simulink model "lvtest3"  (Simulink 7.1)
settings: Solver=ode4  StartTime=0.0  StopTime=90  FixedStep=0.01  RelTol=1e-3
values from neighbouring files (symbols this model uses):
  Ctorque = cq(2:5:102,2:5:182)    [lv_cankaofile.m]    (also in lv_demofile3.m)
  cut_in = 3    [lv_cankaofile.m]    (also in lv_demofile.m; lv_demofile1.m; lv_demofile2.m; lv_demofile3.m)
  cut_out = 25    [lv_cankaofile.m]    (also in lv_demofile.m; lv_demofile1.m; lv_demofile2.m; lv_demofile3.m)
  fs = 50    [lv_cankaofile.m]
  Jem = 90    [lv_cankaofile.m]    (also in lv_demofile.m = 97.5; lv_demofile1.m = 97.5; lv_demofile2.m = 97.5; lv_demofile3.m = 97.5)
  Jwt = 9e7    (= 90000000)    [lv_cankaofile.m]    (also in lv_demofile.m = 3275300; lv_demofile1.m = 3275300; lv_demofile2.m = 3275300; lv_demofile3.m = 3275300)
  K = 83    [lv_cankaofile.m]    (also in lv_demofile.m; lv_demofile1.m = 75.76; lv_demofile2.m; lv_demofile3.m = 75.76)
  Lm = 0.0123    [lv_cankaofile.m]
  Lsgm_r = 0.0126    [lv_cankaofile.m]
  Lsgm_s = 0.0125    [lv_cankaofile.m]
  p = 2    [lv_cankaofile.m]
  R = 40    [lv_cankaofile.m]    (also in lv_demofile.m = 38.5; lv_demofile1.m = 38.75; lv_demofile2.m = 38.5; lv_demofile3.m = 38.5)
  ro_air = 1.225    [lv_cankaofile.m]    (also in lv_demofile.m = 1.2236; lv_demofile1.m; lv_demofile2.m = 1.2236; lv_demofile3.m)
  roughness = 600    [lv_cankaofile.m]    (also in lv_demofile1.m; lv_demofile3.m; lv_demofile4.m; lv_demofile5.m)
  Rr = 0.0041    [lv_cankaofile.m]
  Rs = 0.0043    [lv_cankaofile.m]
  steptime = 0.01    [lv_cankaofile.m]    (also in lv_demofile1.m; lv_demofile3.m; lv_demofile4.m; lv_demofile5.m)
  Tact = 0    [lv_cankaofile.m]    (also in lv_demofile.m; lv_demofile1.m; lv_demofile2.m; lv_demofile3.m)
  turb_int = 12    [lv_cankaofile.m]    (also in lv_demofile1.m; lv_demofile3.m; lv_demofile4.m; lv_demofile5.m)
undefined symbols (not defined in the file or in its folder): PP, u0
libraries: wt_blockset_v3 x2
settings Model: Creator=xc  LastModifiedBy=lv

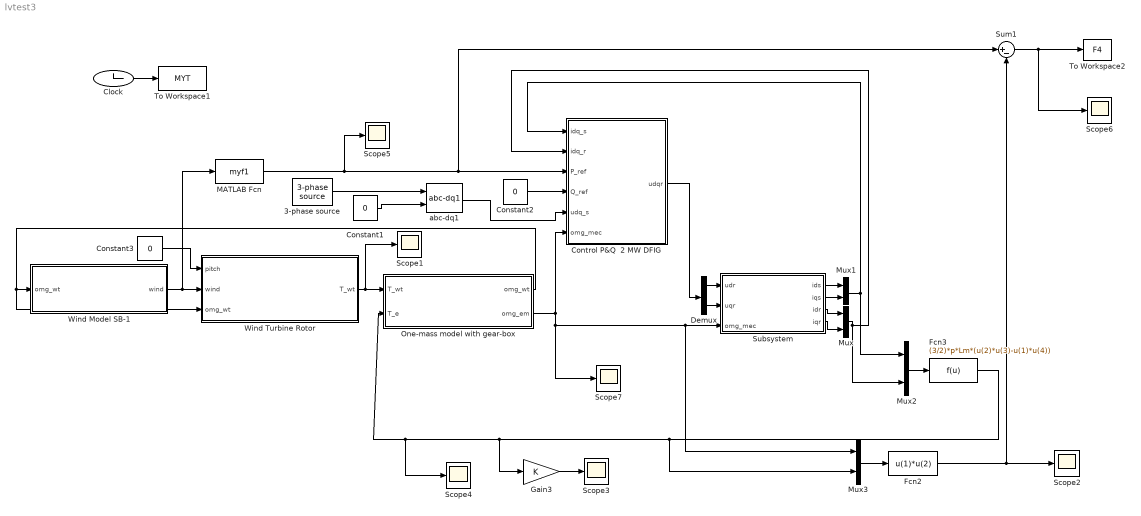
== system lvtest3 ==
  3-phase source : wt_blockset_v3/Grid Models/3-phase source  SystemSampleTime=-1  Uf=220  fs=50
  Clock : Clock
      settings: Decimation=10
  Constant1 : Constant  Value=0  OutDataType=sfix(16)  OutScaling=2^0
  Constant2 : Constant  Value=0  OutDataType=sfix(16)  OutScaling=2^0
  Constant3 : Constant  Value=0  OutDataType=sfix(16)  OutScaling=2^0
  Control P&Q  2 MW DFIG : Subsystem  AncestorBlock="wt_blockset_v3/Control/Control P&Q  2 MW DFIG"  mask(Control P & Q for double feed induction generator){param=[Rs Lsgm_s Rr Lsgm_r Lm], p=p, fs=fs}
      mask prompts: param "Electrical parameters [Rs Lsgm_s Rr Lsgm_r Lm]"; p "Number of pole pais"; fs "Base frequency [Hz]"
      mask help: Control of active and reactive power in synchronous reference frame for DFIG.
      mask init:
      | Rs=param(1); Lsgm_s=param(2); Rr=param(3); Lsgm_r=param(4);
      | Lm=param(5); Lss=Lsgm_s+Lm; Lrr=Lsgm_r+Lm; D=Lss*Lrr-Lm^2;
      | T=D/Lss; Tpr=(Lm^2)/Lss;
      | tau_1=T/Rr;  tau_2=Rr;
      mask Display: disp('Control\nP&Q')
  Demux : Demux  Outputs=2
  Fcn2 : Fcn  Expr=u(1)*u(2)
  Fcn3 : Fcn  Expr=(3/2)*p*Lm*(u(2)*u(3)-u(1)*u(4))
  Gain3 : Gain  Gain=K  ParameterDataType=sfix(16)  ParameterScaling=2^0  OutDataType=sfix(16)  OutScaling=2^0  SaturateOnIntegerOverflow=on  OutDataTypeStr=Inherit: Same as input  ParamDataTypeStr=Inherit: Same as input
  MATLAB Fcn : MATLABFcn  MATLABFcn=myf1
  Mux{,1..3} (4 alike) : Mux  Inputs=2
  One-mass model with gear-box : Subsystem  AncestorBlock=wt_blockset_v3/Mechanical Components/One-mass model with gear-box  mask(Simple Gearbox){Jem=Jem, Jwt=Jwt, K=K, init_speed=1.514}
      mask prompts: Jem "Electric machinery - Moment of inertia [kg m2]"; Jwt "Wind turbine rotor - Moment of inertia [kg*m2]"; K "Gearbox ratio"; init_speed "Initial condition [omg_wt (rad/sec)]"
      mask init:
      | J=Jem*K^2+Jwt;
      mask Display: disp('E M\nGear box')
  Scope{1..7} (7 alike) : Scope
      Scope1 settings: YMin=-2.25e+010  YMax=1.5e+010
      Scope2 settings: TimeRange=90  YMin=-8e+006  YMax=8e+006
      Scope3 settings: YMin=200000  YMax=2.4e+006  SaveName=ScopeData12
      Scope4 settings: YMin=-2.25e+010  YMax=1.5e+010  SaveName=ScopeData6
      Scope5 settings: YMin=-2.25e+010  YMax=1.5e+010  SaveName=ScopeData4
      Scope6 settings: TimeRange=100  YMin=-9e+006  YMax=9e+006  SaveName=ScopeData27
      Scope7 settings: TimeRange=100  YMin=120  YMax=190  SaveName=ScopeData13
  Subsystem : Subsystem
  Sum1 : Sum  Inputs=|+-  OutDataType=sfix(16)  OutScaling=2^0  SaturateOnIntegerOverflow=on  InputSameDT=on  OutDataTypeStr=Inherit: Same as first input
  To Workspace1 : ToWorkspace  VariableName=MYT  SampleTime=-1  SaveFormat=Array
  To Workspace2 : ToWorkspace  VariableName=F4  SampleTime=-1  SaveFormat=Array
  Wind Model SB-1 : Subsystem  AncestorBlock=wt_blockset_v3/Mechanical Components/Wind Model SB-1  TreatAsAtomicUnit=on  mask(Wind Model using Simulink Band-limited white noise generator){D_rotor=2*R, v_mean=10, roughness=roughness, turb_int=turb_int, T_sample=steptime}
      mask prompts: D_rotor "Rotor diameter [m]"; v_mean "Average wind speed [m/sec]"; roughness "Length scale [m]"; turb_int "Turbulence intensity [%]"; T_sample "Sample time [sec]"
      mask help:
      | Implements a rotor wind model developped by RISOE National Laboratory based on Kaimal spectra. The model takes into account the rotational turbulences and the tower shadow.
      | This model uses the built-in band-limited white noise generator from Simulink with different seeds.
      mask init:
      | r = D_rotor/2;
      | sigma = v_mean*turb_int/100;
      | var = sigma^2;
      | c = roughness/(2*pi*v_mean);
      | d = r/v_mean;
      | trans=sigma*sqrt(roughness/v_mean);
      | random=[256, 894, 31];
      mask Display: disp('Wind\nModel\n(SB-1)')
  Wind Turbine Rotor : Subsystem  AncestorBlock=wt_blockset_beta/Mechanical Components/Wind Turbine Rotor  mask(Aerodynamic model for wind turbine){R=R, ro_air=ro_air, cut_in=cut_in, cut_out=cut_out, Tact=Tact}
      mask prompts: R "Blade radius [m]"; ro_air "Air density [kg m3]"; cut_in "Cut in speed [m/sec]"; cut_out "Cut out speed [m/sec]"; Tact "Time constant for pitch actuator [sec]"
      mask init:
      | %cq_table
      mask Display: plot(20,0,120,200,[45,35,35,45,75,75,45],[85,92,108,115,115,85,85],[55,50,70,65],[115,180,190,115],[55,50,70,65],[85,10,20,85],[75,85],[102,102],[75,85],[98,98],[105,85,85,105],[80,85,115,120])
  abc-dq1 : wt_blockset_v3/Electrical Machinery/Simulink Blocks  based Models/Wound Rotor Induction Machine constant parameters/abc-dq1  SystemSampleTime=-1
  wires:
  MATLAB Fcn/1 -> Scope5/1, Sum1/1, Control P&Q  2 MW DFIG/3(P_ref)
  Constant2/1 -> Control P&Q  2 MW DFIG/4(Q_ref)
  Subsystem/1(ids) -> Mux1/1
  Subsystem/2(iqs) -> Mux1/2
  Mux1/1 -> Mux2/1, Control P&Q  2 MW DFIG/1(idq_s)
  Subsystem/3(idr) -> Mux/1
  Subsystem/4(iqr) -> Mux/2
  Mux/1 -> Mux2/2, Control P&Q  2 MW DFIG/2(idq_r)
  Control P&Q  2 MW DFIG/1(udqr) -> Demux/1
  Demux/1 -> Subsystem/1(udr)
  Demux/2 -> Subsystem/2(uqr)
  Wind Turbine Rotor/1(T_wt) -> One-mass model with gear-box/1(T_wt), Scope1/1
  Constant3/1 -> Wind Turbine Rotor/1(pitch)
  Wind Model SB-1/1(wind) -> Wind Turbine Rotor/2(wind), MATLAB Fcn/1
  One-mass model with gear-box/1(omg_wt) -> Wind Model SB-1/1(omg_wt), Wind Turbine Rotor/3(omg_wt)
  Mux2/1 -> Fcn3/1
  Fcn3/1 -> Gain3/1, One-mass model with gear-box/2(T_e), Scope4/1, Mux3/2
  Gain3/1 -> Scope3/1
  Mux3/1 -> Fcn2/1
  Fcn2/1 -> Scope2/1, Sum1/2
  One-mass model with gear-box/2(omg_em) -> Control P&Q  2 MW DFIG/6(omg_mec), Subsystem/3(omg_mec), Mux3/1, Scope7/1
  Clock/1 -> To Workspace1/1
  Sum1/1 -> To Workspace2/1, Scope6/1
  3-phase source/1 -> abc-dq1/1
  Constant1/1 -> abc-dq1/2
  abc-dq1/1 -> Control P&Q  2 MW DFIG/5(udq_s)

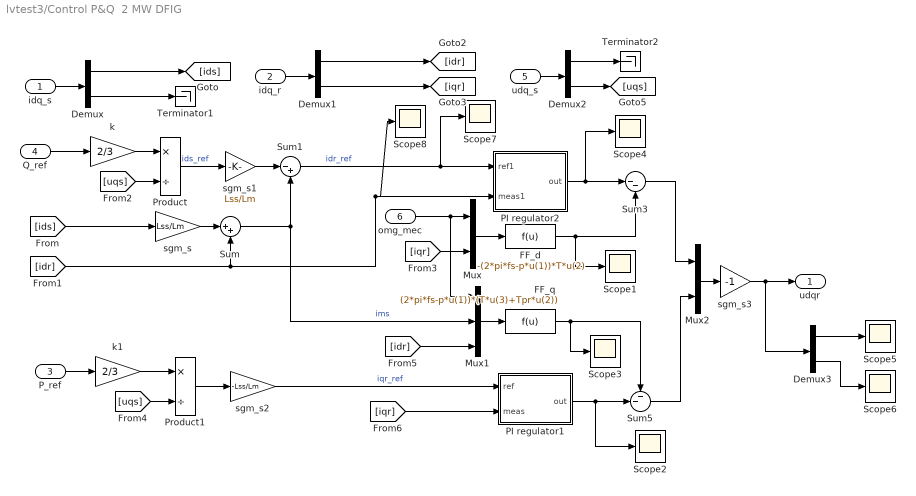
== system lvtest3/Control P&Q  2 MW DFIG ==
  idq_s : Inport  OutDataType=sfix(16)  OutScaling=2^0
  idq_r : Inport  Port=2  OutDataType=sfix(16)  OutScaling=2^0
  P_ref : Inport  Port=3  OutDataType=sfix(16)  OutScaling=2^0
  Q_ref : Inport  Port=4  OutDataType=sfix(16)  OutScaling=2^0
  udq_s : Inport  Port=5  OutDataType=sfix(16)  OutScaling=2^0
  omg_mec : Inport  Port=6  OutDataType=sfix(16)  OutScaling=2^0
  Demux{,1..3} (4 alike) : Demux  Outputs=2
  FF_d : Fcn  Expr=-(2*pi*fs-p*u(1))*T*u(2)
  FF_q : Fcn  Expr=(2*pi*fs-p*u(1))*(T*u(3)+Tpr*u(2))
  Mux : Mux  Inputs=2
  Mux1 : Mux  Inputs=3
  Mux2 : Mux  Inputs=2
  PI regulator1 : Subsystem  mask{K=PP(3), Ti=PP(4), ka=10, maxim=100, init_cond=0}
      mask prompts: K "Proportional Constant"; Ti "Integrate constant"; maxim "Limits"; init_cond "initial"
  PI regulator2 : Subsystem  mask{K=PP(1), Ti=PP(2), init_cond=0}
      mask prompts: K "Proportional Constant"; Ti "Integrate constant"; init_cond "initial"
  Product : Product  Inputs=*/  OutDataType=sfix(16)  OutScaling=2^0  SaturateOnIntegerOverflow=on  InputSameDT=on  OutDataTypeStr=Inherit: Same as first input
  Product1 : Product  Inputs=*/  OutDataType=sfix(16)  OutScaling=2^0  SaturateOnIntegerOverflow=on  InputSameDT=on  OutDataTypeStr=Inherit: Same as first input
  Scope{1..8} (8 alike) : Scope
      Scope1 settings: YMin=-2.25e+010  YMax=1.5e+010  SaveName=ScopeData5
      Scope2 settings: YMin=-2.25e+010  YMax=1.5e+010  SaveName=ScopeData7
      Scope3 settings: YMin=-2.25e+010  YMax=1.5e+010  SaveName=ScopeData3
      Scope4 settings: YMin=-125  YMax=150  SaveName=ScopeData8
      Scope5 settings: YMin=-2.25e+010  YMax=1.5e+010  SaveName=ScopeData9
      Scope6 settings: YMin=-2.25e+010  YMax=1.5e+010  SaveName=ScopeData10
      Scope7 settings: YMin=-2.25e+010  YMax=1.5e+010  SaveName=ScopeData28
      Scope8 settings: YMin=-2.25e+010  YMax=1.5e+010  SaveName=ScopeData29
  Sum : Sum  Inputs=|++  OutDataType=sfix(16)  OutScaling=2^0  SaturateOnIntegerOverflow=on  InputSameDT=on  OutDataTypeStr=Inherit: Same as first input
  Sum1 : Sum  Inputs=|-+  OutDataType=sfix(16)  OutScaling=2^0  SaturateOnIntegerOverflow=on  InputSameDT=on  OutDataTypeStr=Inherit: Same as first input
  Sum3 : Sum  Inputs=|--  OutDataType=sfix(16)  OutScaling=2^0  SaturateOnIntegerOverflow=on  InputSameDT=on  OutDataTypeStr=Inherit: Same as first input
  Sum5 : Sum  Inputs=--|  OutDataType=sfix(16)  OutScaling=2^0  SaturateOnIntegerOverflow=on  InputSameDT=on  OutDataTypeStr=Inherit: Same as first input
  Terminator1 : Terminator
  Terminator2 : Terminator
  k : Gain  Gain=2/3  ParameterDataType=sfix(16)  ParameterScaling=2^0  OutDataType=sfix(16)  OutScaling=2^0  SaturateOnIntegerOverflow=on  OutDataTypeStr=Inherit: Same as input  ParamDataTypeStr=Inherit: Same as input
  k1 : Gain  Gain=2/3  ParameterDataType=sfix(16)  ParameterScaling=2^0  OutDataType=sfix(16)  OutScaling=2^0  SaturateOnIntegerOverflow=on  OutDataTypeStr=Inherit: Same as input  ParamDataTypeStr=Inherit: Same as input
  sgm_s : Gain  Gain=Lss/Lm  ParameterDataType=sfix(16)  ParameterScaling=2^0  OutDataType=sfix(16)  OutScaling=2^0  SaturateOnIntegerOverflow=on  OutDataTypeStr=Inherit: Same as input  ParamDataTypeStr=Inherit: Same as input
  sgm_s1 : Gain  Gain=Lss/Lm  ParameterDataType=sfix(16)  ParameterScaling=2^0  OutDataType=sfix(16)  OutScaling=2^0  SaturateOnIntegerOverflow=on  OutDataTypeStr=Inherit: Same as input  ParamDataTypeStr=Inherit: Same as input
  sgm_s2 : Gain  Gain=-Lss/Lm  ParameterDataType=sfix(16)  ParameterScaling=2^0  OutDataType=sfix(16)  OutScaling=2^0  SaturateOnIntegerOverflow=on  OutDataTypeStr=Inherit: Same as input  ParamDataTypeStr=Inherit: Same as input
  sgm_s3 : Gain  Gain=-1  ParameterDataType=sfix(16)  ParameterScaling=2^0  OutDataType=sfix(16)  OutScaling=2^0  SaturateOnIntegerOverflow=on  OutDataTypeStr=Inherit: Same as input  ParamDataTypeStr=Inherit: Same as input
  udqr : Outport  OutDataType=sfix(16)  OutScaling=2^0
  wires:
  idq_s/1 -> Demux/1
  idq_r/1 -> Demux1/1
  Demux/1 -> [ids]
  Demux/2 -> Terminator1/1
  Demux1/2 -> [iqr]
  [ids] -> sgm_s/1
  sgm_s/1 -> Sum/1
  [idr] -> Sum/2, PI regulator2/2(meas1), Scope8/1
  udq_s/1 -> Demux2/1
  Demux2/1 -> Terminator2/1
  Demux2/2 -> [uqs]
  Q_ref/1 -> k/1
  k/1 -> Product/1
  [uqs] -> Product/2
  Product/1 -> sgm_s1/1  "ids_ref"
  Sum/1 -> Sum1/2, Mux1/2  "ims"
  PI regulator2/1(out) -> Sum3/1, Scope4/1
  omg_mec/1 -> Mux/1, Mux1/1
  Mux/1 -> FF_d/1
  [iqr] -> Mux/2
  Sum3/1 -> Mux2/1
  P_ref/1 -> k1/1
  k1/1 -> Product1/1
  [uqs] -> Product1/2
  Product1/1 -> sgm_s2/1
  sgm_s2/1 -> PI regulator1/1(ref)  "iqr_ref"
  Mux1/1 -> FF_q/1
  PI regulator1/1(out) -> Sum5/2, Scope2/1
  [idr] -> Mux1/3
  Sum5/1 -> Mux2/2
  Mux2/1 -> sgm_s3/1
  sgm_s1/1 -> Sum1/1
  Sum1/1 -> PI regulator2/1(ref1), Scope7/1  "idr_ref"
  FF_d/1 -> Sum3/2, Scope1/1
  [iqr] -> PI regulator1/2(meas)
  FF_q/1 -> Scope3/1, Sum5/1
  Demux1/1 -> [idr]
  Demux3/1 -> Scope5/1
  Demux3/2 -> Scope6/1
  sgm_s3/1 -> udqr/1, Demux3/1

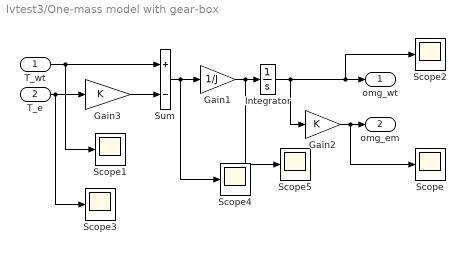
== system lvtest3/One-mass model with gear-box ==
  T_wt : Inport  OutDataType=sfix(16)  OutScaling=2^0
  T_e : Inport  Port=2  OutDataType=sfix(16)  OutScaling=2^0
  Gain1 : Gain  Gain=1/J  ParameterDataType=sfix(16)  ParameterScaling=2^0  OutDataType=sfix(16)  OutScaling=2^0  SaturateOnIntegerOverflow=on  OutDataTypeStr=Inherit: Same as input  ParamDataTypeStr=Inherit: Same as input
  Gain2 : Gain  Gain=K  ParameterDataType=sfix(16)  ParameterScaling=2^0  OutDataType=sfix(16)  OutScaling=2^0  SaturateOnIntegerOverflow=on  OutDataTypeStr=Inherit: Same as input  ParamDataTypeStr=Inherit: Same as input
  Gain3 : Gain  Gain=K  ParameterDataType=sfix(16)  ParameterScaling=2^0  OutDataType=sfix(16)  OutScaling=2^0  SaturateOnIntegerOverflow=on  OutDataTypeStr=Inherit: Same as input  ParamDataTypeStr=Inherit: Same as input
  Integrator : Integrator  InitialCondition=init_speed  UpperSaturationLimit=0.95*2*pi*60  LowerSaturationLimit=0
  Scope{,1..5} (6 alike) : Scope
      Scope settings: TimeRange=10  SaveName=ScopeData20
      Scope1 settings: TimeRange=10  SaveName=ScopeData24
      Scope2 settings: YMin=-2.25e+010  YMax=1.5e+010  SaveName=ScopeData21
      Scope3 settings: TimeRange=10  SaveName=ScopeData25
      Scope4 settings: TimeRange=10  SaveName=ScopeData2
      Scope5 settings: TimeRange=10  SaveName=ScopeData22
  Sum : Sum  Inputs=+-  OutDataType=sfix(16)  OutScaling=2^0  SaturateOnIntegerOverflow=on  InputSameDT=on  OutDataTypeStr=Inherit: Same as first input
  omg_wt : Outport  OutDataType=sfix(16)  OutScaling=2^0  InitialOutput=0
  omg_em : Outport  Port=2  OutDataType=sfix(16)  OutScaling=2^0  InitialOutput=0
  wires:
  Gain3/1 -> Sum/2
  Gain2/1 -> omg_em/1, Scope/1
  Integrator/1 -> Gain2/1, omg_wt/1, Scope2/1
  T_wt/1 -> Sum/1, Scope1/1
  T_e/1 -> Gain3/1, Scope3/1
  Sum/1 -> Gain1/1, Scope4/1
  Gain1/1 -> Integrator/1, Scope5/1

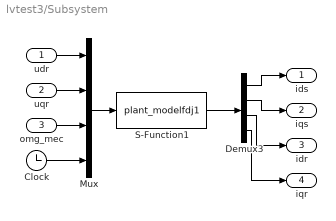
== system lvtest3/Subsystem ==
  udr : Inport
  uqr : Inport  Port=2
  omg_mec : Inport  Port=3
  Clock : Clock
      settings: Decimation=10
  Demux3 : Demux
  Mux : Mux
  S-Function1 : S-Function  FunctionName=plant_modelfdj1  EnableBusSupport=off
  ids : Outport  OutDataType=sfix(16)  OutScaling=2^0  InitialOutput=0
  iqs : Outport  Port=2  OutDataType=sfix(16)  OutScaling=2^0  InitialOutput=0
  idr : Outport  Port=3  OutDataType=sfix(16)  OutScaling=2^0  InitialOutput=0
  iqr : Outport  Port=4  OutDataType=sfix(16)  OutScaling=2^0  InitialOutput=0
  wires:
  Mux/1 -> S-Function1/1
  udr/1 -> Mux/1
  S-Function1/1 -> Demux3/1
  omg_mec/1 -> Mux/3
  uqr/1 -> Mux/2
  Demux3/1 -> ids/1
  Demux3/2 -> iqs/1
  Demux3/3 -> idr/1
  Demux3/4 -> iqr/1
  Clock/1 -> Mux/4

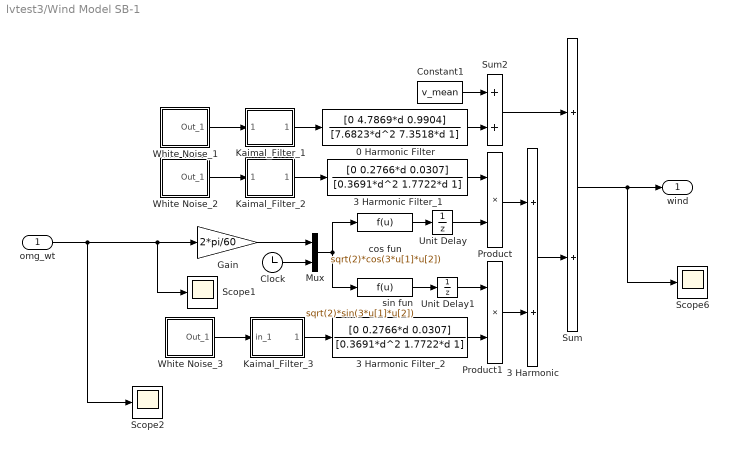
== system lvtest3/Wind Model SB-1 ==
  omg_wt : Inport  OutDataType=sfix(16)  OutScaling=2^0
  0 Harmonic Filter : TransferFcn  Numerator=[0 4.7869*d 0.9904]  Denominator=[7.6823*d^2 7.3518*d 1]
  3 Harmonic : Sum  OutDataType=sfix(16)  OutScaling=2^0  SaturateOnIntegerOverflow=on  InputSameDT=on  OutDataTypeStr=Inherit: Same as first input
  3 Harmonic Filter_1 : TransferFcn  Numerator=[0 0.2766*d 0.0307]  Denominator=[0.3691*d^2 1.7722*d 1]
  3 Harmonic Filter_2 : TransferFcn  Numerator=[0 0.2766*d 0.0307]  Denominator=[0.3691*d^2 1.7722*d 1]
  Clock : Clock
  Constant1 : Constant  Value=v_mean  OutDataType=sfix(16)  OutScaling=2^0
  Gain : Gain  Gain=2*pi/60  ParameterDataType=sfix(16)  ParameterScaling=2^0  OutDataType=sfix(16)  OutScaling=2^0  SaturateOnIntegerOverflow=on  OutDataTypeStr=Inherit: Same as input  ParamDataTypeStr=Inherit: Same as input
  Kaimal_Filter_1 : Subsystem
  Kaimal_Filter_2 : Subsystem
  Kaimal_Filter_3 : Subsystem
  Mux : Mux  Inputs=2
  Product : Product  OutDataType=sfix(16)  OutScaling=2^0  SaturateOnIntegerOverflow=on  InputSameDT=on  OutDataTypeStr=Inherit: Same as first input
  Product1 : Product  OutDataType=sfix(16)  OutScaling=2^0  SaturateOnIntegerOverflow=on  InputSameDT=on  OutDataTypeStr=Inherit: Same as first input
  Scope1 : Scope
      settings: YMin=-2.25e+010  YMax=1.5e+010  SaveName=ScopeData22
  Scope2 : Scope
      settings: YMin=-2.25e+010  YMax=1.5e+010  SaveName=ScopeData20
  Scope6 : Scope
      settings: TimeRange=100  YMin=-9e+006  YMax=9e+006  SaveName=ScopeData39
  Sum : Sum  OutDataType=sfix(16)  OutScaling=2^0  SaturateOnIntegerOverflow=on  InputSameDT=on  OutDataTypeStr=Inherit: Same as first input
  Sum2 : Sum  OutDataType=sfix(16)  OutScaling=2^0  SaturateOnIntegerOverflow=on  InputSameDT=on  OutDataTypeStr=Inherit: Same as first input
  Unit Delay : UnitDelay  SampleTime=T_sample
  Unit Delay1 : UnitDelay  SampleTime=T_sample
  White Noise_1 : Subsystem  mask(Continuous White Noise.){Cov=[1], Ts=T_sample, seed=[random(1)]}
      mask prompts: Cov "Noise Power:"; Ts "Sample Time:"
      mask help:
      | White noise for continuous (s-domain) systems.
      | Band-limited using zero-order-hold.
      mask init:
      | r = rand(1,12); r2 = [r(1),r;r,r(12)]; t =[1:13;1:13];
      mask Help: Implemented using white noise into Zero-Order Hold block. The seed and power can be vectors of the same length to produce a vector of white noise sources. For faster simulation, set sample time to the highest value possible but in accordance with the fastest dynamics of system.
      mask Display: plot(t(:),r2(:))
  White Noise_2 : Subsystem  mask(Continuous White Noise.){@1=[1], @2=T_sample, @3=[random(2)]}
      mask prompts: @1 "Noise Power:"; @2 "Sample Time:"; @3 "Seed"
      mask help:
      | White noise for continuous (s-domain) systems.
      | Band-limited using zero-order-hold.
      mask init:
      | Cov = @1; Ts = @2; seed = @3; r = rand(1,12); r2 = [r(1),r;r,r(12)]; t =[1:13;1:13];
      mask Help: Implemented using white noise into Zero-Order Hold block. The seed and power can be vectors of the same length to produce a vector of white noise sources. For faster simulation, set sample time to the highest value possible but in accordance with the fastest dynamics of system.
      mask Display: plot(t(:),r2(:))
  White Noise_3 : Subsystem  mask(Continuous White Noise.){@1=[1], @2=T_sample, @3=[random(3)]}
      mask prompts: @1 "Noise Power:"; @2 "Sample Time:"; @3 "Seed"
      mask help:
      | White noise for continuous (s-domain) systems.
      | Band-limited using zero-order-hold.
      mask init:
      | Cov = @1; Ts = @2; seed = @3; r = rand(1,12); r2 = [r(1),r;r,r(12)]; t =[1:13;1:13];
      mask Help: Implemented using white noise into Zero-Order Hold block. The seed and power can be vectors of the same length to produce a vector of white noise sources. For faster simulation, set sample time to the highest value possible but in accordance with the fastest dynamics of system.
      mask Display: plot(t(:),r2(:))
  cos fun : Fcn  Expr=sqrt(2)*cos(3*u[1]*u[2])
  sin fun : Fcn  Expr=sqrt(2)*sin(3*u[1]*u[2])
  wind : Outport  OutDataType=sfix(16)  OutScaling=2^0  InitialOutput=[u0]
  wires:
  Clock/1 -> Mux/2
  Unit Delay1/1 -> Product1/1
  Unit Delay/1 -> Product/2
  Gain/1 -> Mux/1
  omg_wt/1 -> Gain/1, Scope1/1, Scope2/1
  Mux/1 -> sin fun/1, cos fun/1
  3 Harmonic Filter_1/1 -> Product/1
  White Noise_3/1(Out_1) -> Kaimal_Filter_3/1(in_1)
  White Noise_2/1(Out_1) -> Kaimal_Filter_2/1(in_1)
  White Noise_1/1(Out_1) -> Kaimal_Filter_1/1(in_1)
  Kaimal_Filter_1/1(out_1) -> 0 Harmonic Filter/1
  Sum/1 -> wind/1, Scope6/1
  Constant1/1 -> Sum2/1
  Sum2/1 -> Sum/1
  0 Harmonic Filter/1 -> Sum2/2
  3 Harmonic/1 -> Sum/2
  3 Harmonic Filter_2/1 -> Product1/2
  Product1/1 -> 3 Harmonic/2
  Product/1 -> 3 Harmonic/1
  sin fun/1 -> Unit Delay1/1
  cos fun/1 -> Unit Delay/1
  Kaimal_Filter_3/1(out_1) -> 3 Harmonic Filter_2/1
  Kaimal_Filter_2/1(out_1) -> 3 Harmonic Filter_1/1

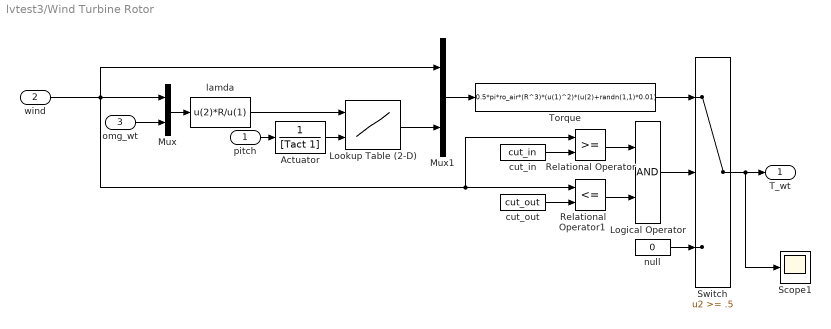
== system lvtest3/Wind Turbine Rotor ==
  pitch : Inport  OutDataType=sfix(16)  OutScaling=2^0
  wind : Inport  Port=2  OutDataType=sfix(16)  OutScaling=2^0
  omg_wt : Inport  Port=3  OutDataType=sfix(16)  OutScaling=2^0
  Actuator : TransferFcn  Denominator=[Tact 1]
  Logical Operator : Logic
  Lookup Table (2-D) : Lookup2D  RowIndex=[0:1:20]  ColumnIndex=[-90:5:90]  Table=Ctorque  OutDataType=sfix(16)  OutScaling=2^0
  Mux : Mux  Inputs=2
  Mux1 : Mux  Inputs=2
  Relational Operator : RelationalOperator  InputSameDT=on
  Relational Operator1 : RelationalOperator  Operator=<=  InputSameDT=on
  Scope1 : Scope
      settings: TimeRange=20  YMin=-1500000  YMax=1500000  SaveName=ScopeData19
  Switch : Switch  Threshold=.5  SaturateOnIntegerOverflow=on  InputSameDT=on
  Torque : Fcn  Expr=0.5*pi*ro_air*(R^3)*(u(1)^2)*(u(2)+randn(1,1)*0.01)
  cut_in : Constant  Value=cut_in  OutDataType=sfix(16)  OutScaling=2^0
  cut_out : Constant  Value=cut_out  OutDataType=sfix(16)  OutScaling=2^0
  lamda : Fcn  Expr=u(2)*R/u(1)
  null : Constant  Value=0  OutDataType=sfix(16)  OutScaling=2^0
  T_wt : Outport
  wires:
  Actuator/1 -> Lookup Table (2-D)/2
  Mux/1 -> lamda/1
  Mux1/1 -> Torque/1
  omg_wt/1 -> Mux/2
  cut_in/1 -> Relational Operator/2
  cut_out/1 -> Relational Operator1/2
  Relational Operator1/1 -> Logical Operator/2
  Relational Operator/1 -> Logical Operator/1
  Switch/1 -> T_wt/1, Scope1/1
  Torque/1 -> Switch/1
  null/1 -> Switch/3
  Logical Operator/1 -> Switch/2
  wind/1 -> Mux/1, Relational Operator/1, Relational Operator1/1, Mux1/1
  Lookup Table (2-D)/1 -> Mux1/2
  lamda/1 -> Lookup Table (2-D)/1
  pitch/1 -> Actuator/1

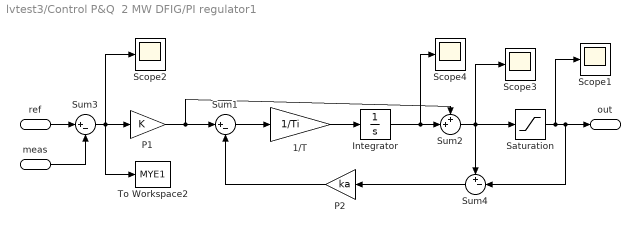
== system lvtest3/Control P&Q  2 MW DFIG/PI regulator1 ==
  ref : Inport  OutDataType=sfix(16)  OutScaling=2^0
  meas : Inport  Port=2  OutDataType=sfix(16)  OutScaling=2^0
  1/T : Gain  Gain=1/Ti  ParameterDataType=sfix(16)  ParameterScaling=2^0  OutDataType=sfix(16)  OutScaling=2^0  SaturateOnIntegerOverflow=on  OutDataTypeStr=Inherit: Same as input  ParamDataTypeStr=Inherit: Same as input
  Integrator : Integrator  InitialCondition=init_cond
  P1 : Gain  Gain=K  ParameterDataType=sfix(16)  ParameterScaling=2^0  OutDataType=sfix(16)  OutScaling=2^0  SaturateOnIntegerOverflow=on  OutDataTypeStr=Inherit: Same as input  ParamDataTypeStr=Inherit: Same as input
  P2 : Gain  Orientation=left  Gain=ka  ParameterDataType=sfix(16)  ParameterScaling=2^0  OutDataType=sfix(16)  OutScaling=2^0  SaturateOnIntegerOverflow=on  OutDataTypeStr=Inherit: Same as input  ParamDataTypeStr=Inherit: Same as input
  Saturation : Saturate  UpperLimit=maxim  LowerLimit=-maxim
  Scope{1..4} (4 alike) : Scope
      Scope1 settings: YMin=-45000  YMax=55000  SaveName=ScopeData30
      Scope2 settings: YMin=-2.25e+010  YMax=1.5e+010  SaveName=ScopeData18
      Scope3 settings: YMin=-2.25e+010  YMax=1.5e+010  SaveName=ScopeData31
      Scope4 settings: YMin=-2.25e+010  YMax=1.5e+010  SaveName=ScopeData34
  Sum1 : Sum  Inputs=|+-  OutDataType=sfix(16)  OutScaling=2^0  SaturateOnIntegerOverflow=on  InputSameDT=on  OutDataTypeStr=Inherit: Same as first input
  Sum2 : Sum  Inputs=++|  OutDataType=sfix(16)  OutScaling=2^0  SaturateOnIntegerOverflow=on  InputSameDT=on  OutDataTypeStr=Inherit: Same as first input
  Sum3 : Sum  Inputs=|+-  OutDataType=sfix(16)  OutScaling=2^0  SaturateOnIntegerOverflow=on  InputSameDT=on  OutDataTypeStr=Inherit: Same as first input
  Sum4 : Sum  Orientation=left  Inputs=+-|  OutDataType=sfix(16)  OutScaling=2^0  SaturateOnIntegerOverflow=on  InputSameDT=on  OutDataTypeStr=Inherit: Same as first input
  To Workspace2 : ToWorkspace  VariableName=MYE1  SampleTime=-1  SaveFormat=Array
  out : Outport  OutDataType=sfix(16)  OutScaling=2^0  InitialOutput=0
  wires:
  Sum2/1 -> Scope3/1, Sum4/1, Saturation/1
  meas/1 -> Sum3/2
  P1/1 -> Sum2/1, Sum1/1
  ref/1 -> Sum3/1
  Sum3/1 -> P1/1, To Workspace2/1, Scope2/1
  1/T/1 -> Integrator/1
  Integrator/1 -> Sum2/2, Scope4/1
  Sum1/1 -> 1/T/1
  P2/1 -> Sum1/2
  Sum4/1 -> P2/1
  Saturation/1 -> Scope1/1, Sum4/2, out/1

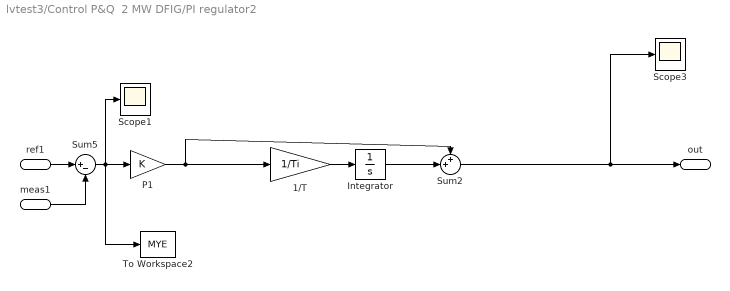
== system lvtest3/Control P&Q  2 MW DFIG/PI regulator2 ==
  ref1 : Inport  OutDataType=sfix(16)  OutScaling=2^0
  meas1 : Inport  Port=2  OutDataType=sfix(16)  OutScaling=2^0
  1/T : Gain  Gain=1/Ti  ParameterDataType=sfix(16)  ParameterScaling=2^0  OutDataType=sfix(16)  OutScaling=2^0  SaturateOnIntegerOverflow=on  OutDataTypeStr=Inherit: Same as input  ParamDataTypeStr=Inherit: Same as input
  Integrator : Integrator  InitialCondition=init_cond
  P1 : Gain  Gain=K  ParameterDataType=sfix(16)  ParameterScaling=2^0  OutDataType=sfix(16)  OutScaling=2^0  SaturateOnIntegerOverflow=on  OutDataTypeStr=Inherit: Same as input  ParamDataTypeStr=Inherit: Same as input
  Scope1 : Scope
      settings: YMin=-4000  YMax=4000  SaveName=ScopeData16
  Scope3 : Scope
      settings: YMin=-7500  YMax=17500  SaveName=ScopeData38
  Sum2 : Sum  Inputs=++|  OutDataType=sfix(16)  OutScaling=2^0  SaturateOnIntegerOverflow=on  InputSameDT=on  OutDataTypeStr=Inherit: Same as first input
  Sum5 : Sum  Inputs=|+-  OutDataType=sfix(16)  OutScaling=2^0  SaturateOnIntegerOverflow=on  InputSameDT=on  OutDataTypeStr=Inherit: Same as first input
  To Workspace2 : ToWorkspace  VariableName=MYE  SampleTime=-1  SaveFormat=Array
  out : Outport  OutDataType=sfix(16)  OutScaling=2^0  InitialOutput=0
  wires:
  Sum2/1 -> out/1, Scope3/1
  P1/1 -> Sum2/1, 1/T/1
  Sum5/1 -> P1/1, To Workspace2/1, Scope1/1
  1/T/1 -> Integrator/1
  Integrator/1 -> Sum2/2
  meas1/1 -> Sum5/2
  ref1/1 -> Sum5/1

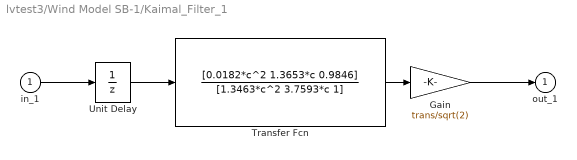
== system lvtest3/Wind Model SB-1/Kaimal_Filter_1 ==
  in_1 : Inport  OutDataType=sfix(16)  OutScaling=2^0
  Gain : Gain  Gain=trans/sqrt(2)  ParameterDataType=sfix(16)  ParameterScaling=2^0  OutDataType=sfix(16)  OutScaling=2^0  SaturateOnIntegerOverflow=on  OutDataTypeStr=Inherit: Same as input  ParamDataTypeStr=Inherit: Same as input
  Transfer Fcn : TransferFcn  Numerator=[0.0182*c^2 1.3653*c 0.9846]  Denominator=[1.3463*c^2 3.7593*c 1]
  Unit Delay : UnitDelay  SampleTime=T_sample
  out_1 : Outport  OutDataType=sfix(16)  OutScaling=2^0
  wires:
  Transfer Fcn/1 -> Gain/1
  in_1/1 -> Unit Delay/1
  Gain/1 -> out_1/1
  Unit Delay/1 -> Transfer Fcn/1

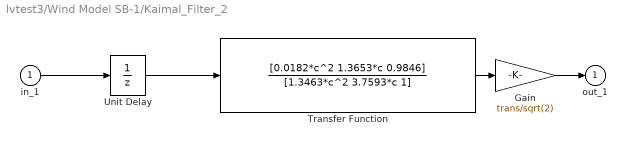
== system lvtest3/Wind Model SB-1/Kaimal_Filter_2 ==
  in_1 : Inport  OutDataType=sfix(16)  OutScaling=2^0
  Gain : Gain  Gain=trans/sqrt(2)  ParameterDataType=sfix(16)  ParameterScaling=2^0  OutDataType=sfix(16)  OutScaling=2^0  SaturateOnIntegerOverflow=on  OutDataTypeStr=Inherit: Same as input  ParamDataTypeStr=Inherit: Same as input
  Transfer Function : TransferFcn  Numerator=[0.0182*c^2 1.3653*c 0.9846]  Denominator=[1.3463*c^2 3.7593*c 1]
  Unit Delay : UnitDelay  SampleTime=T_sample
  out_1 : Outport  OutDataType=sfix(16)  OutScaling=2^0
  wires:
  Transfer Function/1 -> Gain/1
  in_1/1 -> Unit Delay/1
  Gain/1 -> out_1/1
  Unit Delay/1 -> Transfer Function/1

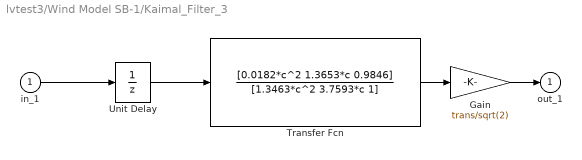
== system lvtest3/Wind Model SB-1/Kaimal_Filter_3 ==
  in_1 : Inport  OutDataType=sfix(16)  OutScaling=2^0
  Gain : Gain  Gain=trans/sqrt(2)  ParameterDataType=sfix(16)  ParameterScaling=2^0  OutDataType=sfix(16)  OutScaling=2^0  SaturateOnIntegerOverflow=on  OutDataTypeStr=Inherit: Same as input  ParamDataTypeStr=Inherit: Same as input
  Transfer Fcn : TransferFcn  Numerator=[0.0182*c^2 1.3653*c 0.9846]  Denominator=[1.3463*c^2 3.7593*c 1]
  Unit Delay : UnitDelay  SampleTime=T_sample
  out_1 : Outport  OutDataType=sfix(16)  OutScaling=2^0
  wires:
  Transfer Fcn/1 -> Gain/1
  in_1/1 -> Unit Delay/1
  Gain/1 -> out_1/1
  Unit Delay/1 -> Transfer Fcn/1

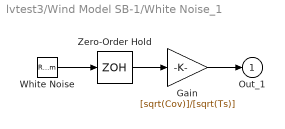
== system lvtest3/Wind Model SB-1/White Noise_1 ==
  Gain : Gain  Gain=[sqrt(Cov)]/[sqrt(Ts)]  ParameterDataType=sfix(16)  ParameterScaling=2^0  OutDataType=sfix(16)  OutScaling=2^0  SaturateOnIntegerOverflow=on  OutDataTypeStr=Inherit: Same as input  ParamDataTypeStr=Inherit: Same as input
  White Noise : RandomNumber  Seed=seed  SampleTime=Ts
  Zero-Order Hold : ZeroOrderHold  SampleTime=Ts
  Out_1 : Outport  OutDataType=sfix(16)  OutScaling=2^0
  wires:
  Zero-Order Hold/1 -> Gain/1
  Gain/1 -> Out_1/1
  White Noise/1 -> Zero-Order Hold/1

== system lvtest3/Wind Model SB-1/White Noise_2 ==
  Gain : Gain  Gain=[sqrt(Cov)]/[sqrt(Ts)]  ParameterDataType=sfix(16)  ParameterScaling=2^0  OutDataType=sfix(16)  OutScaling=2^0  SaturateOnIntegerOverflow=on  OutDataTypeStr=Inherit: Same as input  ParamDataTypeStr=Inherit: Same as input
  White Noise : RandomNumber  Seed=seed  SampleTime=Ts
  Zero-Order Hold : ZeroOrderHold  SampleTime=Ts
  Out_1 : Outport  OutDataType=sfix(16)  OutScaling=2^0
  wires:
  Zero-Order Hold/1 -> Gain/1
  Gain/1 -> Out_1/1
  White Noise/1 -> Zero-Order Hold/1

== system lvtest3/Wind Model SB-1/White Noise_3 ==
  Gain : Gain  Gain=[sqrt(Cov)]/[sqrt(Ts)]  ParameterDataType=sfix(16)  ParameterScaling=2^0  OutDataType=sfix(16)  OutScaling=2^0  SaturateOnIntegerOverflow=on  OutDataTypeStr=Inherit: Same as input  ParamDataTypeStr=Inherit: Same as input
  White Noise : RandomNumber  Seed=seed  SampleTime=Ts
  Zero-Order Hold : ZeroOrderHold  SampleTime=Ts
  Out_1 : Outport  OutDataType=sfix(16)  OutScaling=2^0
  wires:
  Zero-Order Hold/1 -> Gain/1
  Gain/1 -> Out_1/1
  White Noise/1 -> Zero-Order Hold/1
